simulink model "model_NNMPC_control"  (R2025a)
settings: Solver=ode4  StartTime=0.0  StopTime=100  FixedStep=1  RelTol=1e-4
values from neighbouring files (symbols this model uses):
  q = 0.015    [init_params.m]
  T0 = 320    [init_params.m]
  Tc0 = 298    [init_params.m]
undefined symbols (not defined in the file or in its folder): compactSVM
settings Model: Creator=thapl  LastModifiedBy=thapl
settings DataIOCC: SaveFormat=Array
settings OptimizationCC: ReuseModelBlockBuffer=off
settings RTWCC: GPUComputeCapability=3.5

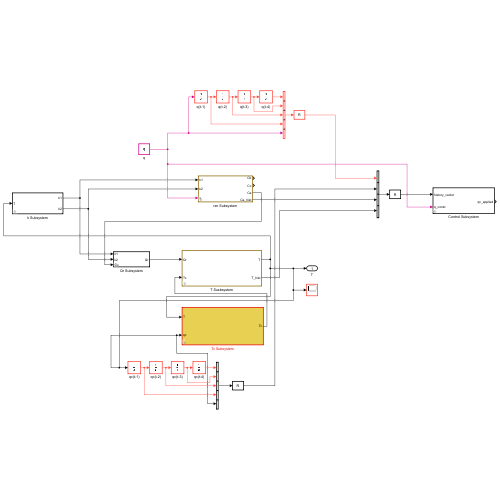
[thumbnail: Simulink's stored preview of the top-level diagram]
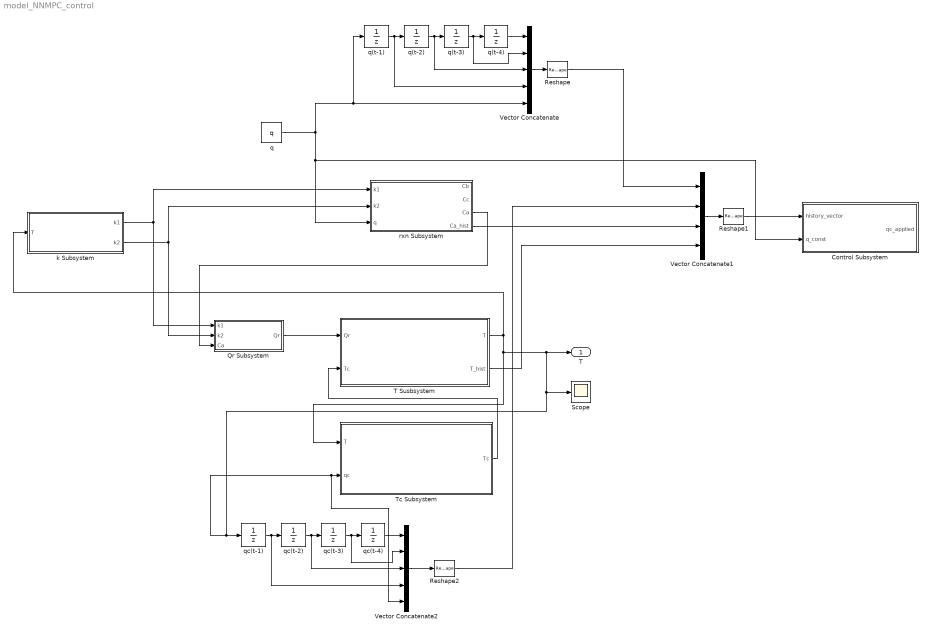
== system model_NNMPC_control ==
  Control Subsystem : Subsystem  mask{T_sp=310}
  Qr Subsystem : Subsystem  mask{V=0.23, dH1=-8.6e4, dH2=-1.82e4}
      mask prompts: V "Reactor Volume (V)"; dH1 "Enthapy of Rxn1 (dH1)"; dH2 "Enthalpy of Rxn2 (dH2)"
  Reshape : Reshape  OutputDimensionality=Customize  OutputDimensions=[1,5]
  Reshape1 : Reshape  OutputDimensionality=Customize  OutputDimensions=[1,20]
  Reshape2 : Reshape  OutputDimensionality=Customize  OutputDimensions=[1,5]
  Scope : Scope
      settings: ActiveDisplayYMinimum=303.48557  ActiveDisplayYMaximum=304.49086
  T Susbsystem : Subsystem  mask{q=0.015, V=0.23, Tf=311, A=1.51, u=42.8, rho=1020, Cp=4.02}
      mask prompts: q "Reactor Flow rate (q)"; V "Reactor Volume (V)"; Tf "Inlet Fluid Temp (Tf)"; A "Contact Area (A)"; u "HTC (u)"; rho "Fluid Density (rho)"; Cp "Specific Heat capactiy (Cp)"
  Tc Subsystem : Subsystem  mask{Vc=0.21, Tcf=292, A=1.51, u=42.8, Cpc=4.182, rhoc=998}
      mask prompts: Vc "Jacket Volume (Vc)"; Tcf "Inlet Cooling Fluid Tempreture (Tcf)"; A "Contact Area (A)"; u "HTC"; Cpc "Specidic Heat Capacity of cooling fluid (Cpc)"; rhoc "Cooling Fluid Density (rhoc)"
  Vector Concatenate : Concatenate  NumInputs=5
  Vector Concatenate1 : Concatenate  NumInputs=4
  Vector Concatenate2 : Concatenate  NumInputs=5
  k Subsystem : Subsystem
      mask DialogControl Control2 Prompt: Text
  q : Constant  Value=q
  q(t-1) : UnitDelay  SampleTime=-1  HasFrameUpgradeWarning=on
  q(t-2) : UnitDelay  SampleTime=-1  HasFrameUpgradeWarning=on
  q(t-3) : UnitDelay  SampleTime=-1  HasFrameUpgradeWarning=on
  q(t-4) : UnitDelay  SampleTime=-1  HasFrameUpgradeWarning=on
  qc(t-1) : UnitDelay  SampleTime=-1  HasFrameUpgradeWarning=on
  qc(t-2) : UnitDelay  SampleTime=-1  HasFrameUpgradeWarning=on
  qc(t-3) : UnitDelay  SampleTime=-1  HasFrameUpgradeWarning=on
  qc(t-4) : UnitDelay  SampleTime=-1  HasFrameUpgradeWarning=on
  rxn Subsystem : Subsystem
      mask DialogControl Control2 Prompt: Reactor
  T : Outport
  wires:
  Tc Subsystem/1(Tc) -> T Susbsystem/2(Tc)
  Qr Subsystem/1(Qr) -> T Susbsystem/1(Qr)
  rxn Subsystem/3(Ca) -> Qr Subsystem/3(Ca)
  k Subsystem/1(k1) -> rxn Subsystem/1(k1), Qr Subsystem/1(k1)
  k Subsystem/2(k2) -> rxn Subsystem/2(k2), Qr Subsystem/2(k2)
  qc(t-2)/1 -> Vector Concatenate2/3, qc(t-3)/1
  qc(t-4)/1 -> Vector Concatenate2/1
  Vector Concatenate2/1 -> Reshape2/1
  qc(t-1)/1 -> Vector Concatenate2/4, qc(t-2)/1
  qc(t-3)/1 -> Vector Concatenate2/2, qc(t-4)/1
  q/1 -> Control Subsystem/2(q_const), rxn Subsystem/3(q), Vector Concatenate/5, q(t-1)/1
  q(t-3)/1 -> Vector Concatenate/2, q(t-4)/1
  q(t-1)/1 -> Vector Concatenate/4, q(t-2)/1
  q(t-4)/1 -> Vector Concatenate/1
  q(t-2)/1 -> Vector Concatenate/3, q(t-3)/1
  Vector Concatenate/1 -> Reshape/1
  rxn Subsystem/4(Ca_hist) -> Vector Concatenate1/3
  Vector Concatenate1/1 -> Reshape1/1
  T Susbsystem/2(T_hist) -> Vector Concatenate1/4
  Reshape/1 -> Vector Concatenate1/1
  Reshape1/1 -> Control Subsystem/1(history_vector)
  Reshape2/1 -> Vector Concatenate1/2
  T Susbsystem/1(T) -> Vector Concatenate2/5, Tc Subsystem/2(qc), qc(t-1)/1, Scope/1, T/1, Tc Subsystem/1(T), k Subsystem/1(T)

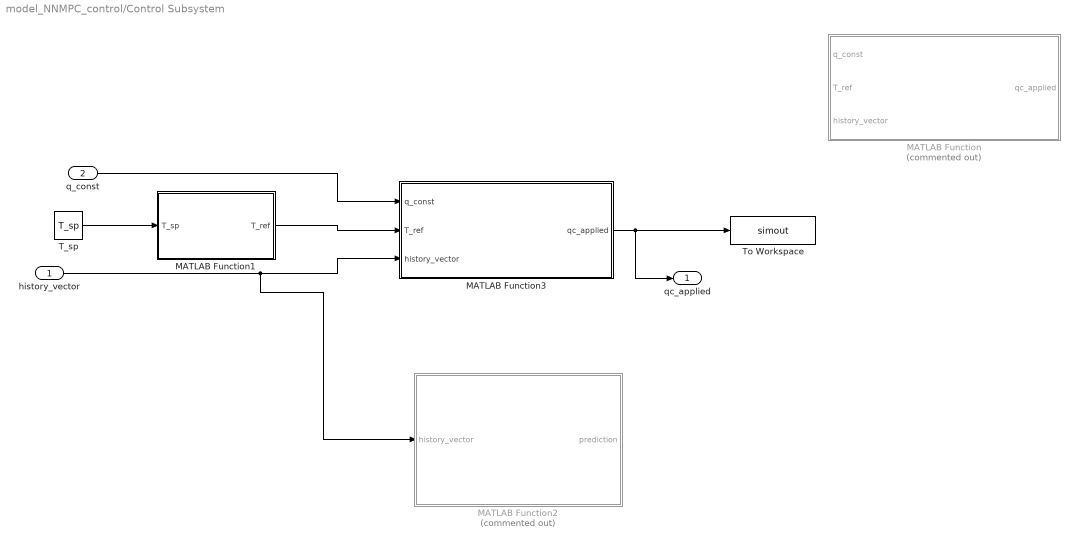
== system model_NNMPC_control/Control Subsystem ==
  history_vector : Inport
  q_const : Inport  Port=2
  MATLAB Function : MATLAB Function  Commented=on  TreatAsAtomicUnit=on  mask{model=compactSVM}
  MATLAB Function1 : MATLAB Function  TreatAsAtomicUnit=on
  MATLAB Function2 : MATLAB Function  Commented=on  TreatAsAtomicUnit=on
  MATLAB Function3 : MATLAB Function  TreatAsAtomicUnit=on
  T_sp : Constant  Value=T_sp
  To Workspace : ToWorkspace  VariableName=simout  SampleTime=-1
      settings: Save2DSignal=2-D array (concatenate along first dimension)
  qc_applied : Outport
  wires:
  T_sp/1 -> MATLAB Function1/1(T_sp)
  history_vector/1 -> MATLAB Function3/3(history_vector), MATLAB Function2/1(history_vector)
  q_const/1 -> MATLAB Function3/1(q_const)
  MATLAB Function1/1(T_ref) -> MATLAB Function3/2(T_ref)
  MATLAB Function3/1(qc_applied) -> qc_applied/1, To Workspace/1

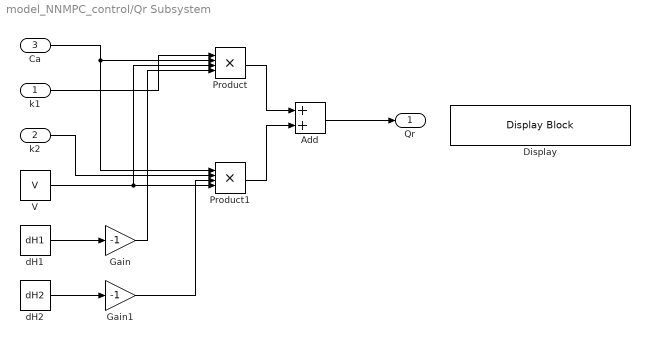
== system model_NNMPC_control/Qr Subsystem ==
  k1 : Inport
  k2 : Inport  Port=2
  Ca : Inport  Port=3
  Add : Sum
  Display : DisplayBlock  LabelPosition=Hide  Transparency=1  GridColor=[0.502, 0.502, 0.502]
  Gain : Gain  Gain=-1
  Gain1 : Gain  Gain=-1
  Product : Product  Inputs=4
  Product1 : Product  Inputs=4
  V : Constant  Value=V
  dH1 : Constant  Value=dH1
  dH2 : Constant  Value=dH2
  Qr : Outport
  wires:
  dH1/1 -> Gain/1
  dH2/1 -> Gain1/1
  k1/1 -> Product/1
  V/1 -> Product1/4, Product/3
  Gain/1 -> Product/4
  Ca/1 -> Product1/1, Product/2
  k2/1 -> Product1/2
  Gain1/1 -> Product1/3
  Product/1 -> Add/1
  Product1/1 -> Add/2
  Add/1 -> Qr/1

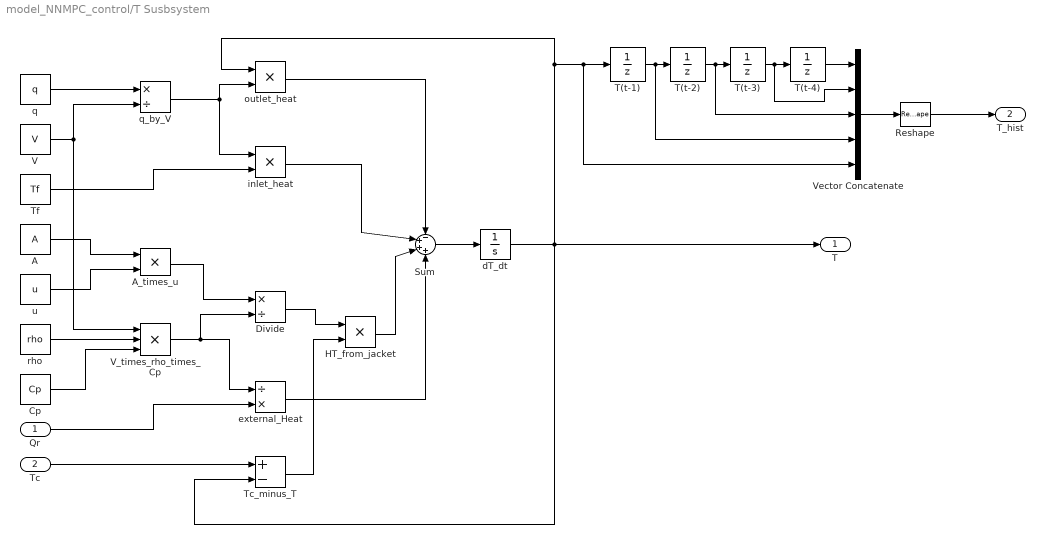
== system model_NNMPC_control/T Susbsystem ==
  Qr : Inport
  Tc : Inport  Port=2
  A : Constant  Value=A
  A_times_u : Product
  Cp : Constant  Value=Cp
  Divide : Product  Inputs=*/
  HT_from_jacket : Product
  Reshape : Reshape  OutputDimensionality=Customize  OutputDimensions=[1,5]
  Sum : Sum  Inputs=-+++
  T(t-1) : UnitDelay  SampleTime=-1  HasFrameUpgradeWarning=on
  T(t-2) : UnitDelay  SampleTime=-1  HasFrameUpgradeWarning=on
  T(t-3) : UnitDelay  SampleTime=-1  HasFrameUpgradeWarning=on
  T(t-4) : UnitDelay  SampleTime=-1  HasFrameUpgradeWarning=on
  Tc_minus_T : Sum  Inputs=+-
  Tf : Constant  Value=Tf
  V : Constant  Value=V
  V_times_rho_times_Cp : Product  Inputs=3
  Vector Concatenate : Concatenate  NumInputs=5
  dT_dt : Integrator  InitialCondition=T0
  external_Heat : Product  Inputs=/*
  inlet_heat : Product
  outlet_heat : Product
  q : Constant  Value=q
  q_by_V : Product  Inputs=*/
  rho : Constant  Value=rho
  u : Constant  Value=u
  T : Outport
  T_hist : Outport  Port=2
  wires:
  q/1 -> q_by_V/1
  V/1 -> V_times_rho_times_Cp/1, q_by_V/2
  q_by_V/1 -> outlet_heat/2, inlet_heat/1
  Tf/1 -> inlet_heat/2
  A/1 -> A_times_u/1
  u/1 -> A_times_u/2
  rho/1 -> V_times_rho_times_Cp/2
  Cp/1 -> V_times_rho_times_Cp/3
  A_times_u/1 -> Divide/1
  V_times_rho_times_Cp/1 -> external_Heat/1, Divide/2
  Divide/1 -> HT_from_jacket/1
  Tc_minus_T/1 -> HT_from_jacket/2
  Qr/1 -> external_Heat/2
  outlet_heat/1 -> Sum/1
  inlet_heat/1 -> Sum/2
  HT_from_jacket/1 -> Sum/3
  external_Heat/1 -> Sum/4
  Sum/1 -> dT_dt/1
  Tc/1 -> Tc_minus_T/1
  dT_dt/1 -> Vector Concatenate/5, T(t-1)/1, outlet_heat/1, T/1, Tc_minus_T/2
  T(t-3)/1 -> Vector Concatenate/2, T(t-4)/1
  T(t-1)/1 -> Vector Concatenate/4, T(t-2)/1
  T(t-4)/1 -> Vector Concatenate/1
  T(t-2)/1 -> Vector Concatenate/3, T(t-3)/1
  Vector Concatenate/1 -> Reshape/1
  Reshape/1 -> T_hist/1

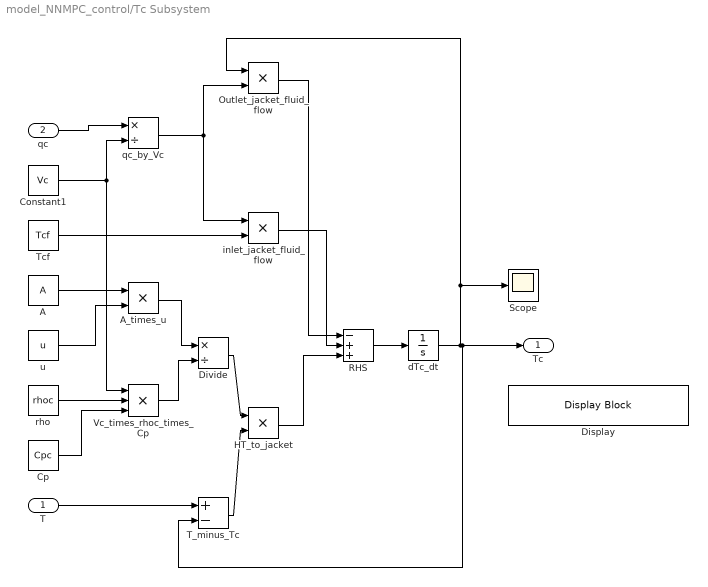
== system model_NNMPC_control/Tc Subsystem ==
  T : Inport
  qc : Inport  Port=2
  A : Constant  Value=A
  A_times_u : Product
  Constant1 : Constant  Value=Vc
  Cp : Constant  Value=Cpc
  Display : DisplayBlock  LabelPosition=Hide  Transparency=1  GridColor=[0.502, 0.502, 0.502]
  Divide : Product  Inputs=*/
  HT_to_jacket : Product
  Outlet_jacket_fluid_flow : Product
  RHS : Sum  Inputs=-++
  Scope : Scope
      settings: ActiveDisplayYMinimum=291.10857  ActiveDisplayYMaximum=300.98794  DataLoggingVariableName=ScopeData3
  T_minus_Tc : Sum  Inputs=+-
  Tcf : Constant  Value=Tcf
  Vc_times_rhoc_times_Cp : Product  Inputs=3
  dTc_dt : Integrator  InitialCondition=Tc0
  inlet_jacket_fluid_flow : Product
  qc_by_Vc : Product  Inputs=*/
  rho : Constant  Value=rhoc
  u : Constant  Value=u
  Tc : Outport
  wires:
  qc/1 -> qc_by_Vc/1
  Constant1/1 -> Vc_times_rhoc_times_Cp/1, qc_by_Vc/2
  qc_by_Vc/1 -> Outlet_jacket_fluid_flow/2, inlet_jacket_fluid_flow/1
  Tcf/1 -> inlet_jacket_fluid_flow/2
  A/1 -> A_times_u/1
  u/1 -> A_times_u/2
  rho/1 -> Vc_times_rhoc_times_Cp/2
  Cp/1 -> Vc_times_rhoc_times_Cp/3
  A_times_u/1 -> Divide/1
  Vc_times_rhoc_times_Cp/1 -> Divide/2
  T/1 -> T_minus_Tc/1
  Divide/1 -> HT_to_jacket/1
  T_minus_Tc/1 -> HT_to_jacket/2
  HT_to_jacket/1 -> RHS/3
  inlet_jacket_fluid_flow/1 -> RHS/2
  RHS/1 -> dTc_dt/1
  dTc_dt/1 -> Scope/1, Outlet_jacket_fluid_flow/1, Tc/1, T_minus_Tc/2
  Outlet_jacket_fluid_flow/1 -> RHS/1

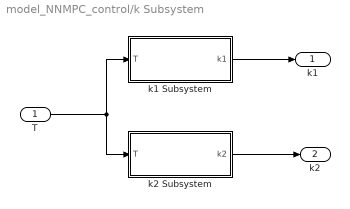
== system model_NNMPC_control/k Subsystem ==
  T : Inport
  k1 Subsystem : Subsystem  mask{R=8.314, k10=1.55e11, Ea1=9850*8.314}
      mask prompts: R "Universal Gas Constant(R)"; k10 "Pre exponential factor(k10)"; Ea1 "Actvation Energy(Ea1)"
  k2 Subsystem : Subsystem  mask{R=8.314, k20=4.55e25, Ea2=22019*8.314}
      mask prompts: R "Universal Gas Constant(R)"; k20 "Pre exponential factor(k10)"; Ea2 "Actvation Energy(Ea1)"
  k1 : Outport
  k2 : Outport  Port=2
  wires:
  k2 Subsystem/1(k2) -> k2/1
  T/1 -> k2 Subsystem/1(T), k1 Subsystem/1(T)
  k1 Subsystem/1(k1) -> k1/1

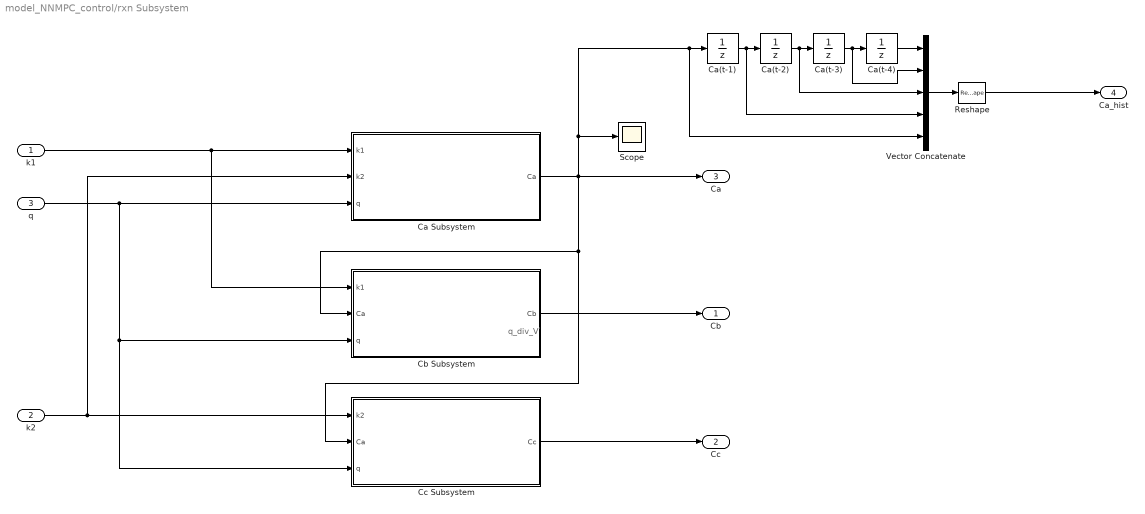
== system model_NNMPC_control/rxn Subsystem ==
  note: q_div_V
  k1 : Inport
  k2 : Inport  Port=2
  q : Inport  Port=3
  Ca Subsystem : Subsystem  mask{V=0.23, Caf=4.22}
      mask prompts: V "Reactor Volume(V)"; Caf "Feed Conc (Caf)"
  Ca(t-1) : UnitDelay  SampleTime=-1  HasFrameUpgradeWarning=on
  Ca(t-2) : UnitDelay  SampleTime=-1  HasFrameUpgradeWarning=on
  Ca(t-3) : UnitDelay  SampleTime=-1  HasFrameUpgradeWarning=on
  Ca(t-4) : UnitDelay  SampleTime=-1  HasFrameUpgradeWarning=on
  Cb Subsystem : Subsystem  mask{V=0.23, Cbf=0}
      mask prompts: V "Reactor Volume(V)"; Cbf "Feed Conc (Cbf)"
  Cc Subsystem : Subsystem  mask{V=0.23, Ccf=0}
      mask prompts: V "Reactor Volume(V)"; Ccf "Feed Conc (Ccf)"
  Reshape : Reshape  OutputDimensionality=Customize  OutputDimensions=[1,5]
  Scope : Scope
      settings: ActiveDisplayYMinimum=3.8625867142774011  ActiveDisplayYMaximum=4.259712587302511
  Vector Concatenate : Concatenate  NumInputs=5
  Cb : Outport
  Cc : Outport  Port=2
  Ca : Outport  Port=3
  Ca_hist : Outport  Port=4
  wires:
  k1/1 -> Cb Subsystem/1(k1), Ca Subsystem/1(k1)
  Cc Subsystem/1(Cc) -> Cc/1
  Cb Subsystem/1(Cb) -> Cb/1
  k2/1 -> Cc Subsystem/1(k2), Ca Subsystem/2(k2)
  q/1 -> Cc Subsystem/3(q), Cb Subsystem/3(q), Ca Subsystem/3(q)
  Ca Subsystem/1(Ca) -> Cc Subsystem/2(Ca), Cb Subsystem/2(Ca), Vector Concatenate/5, Ca(t-1)/1, Scope/1, Ca/1
  Ca(t-3)/1 -> Vector Concatenate/2, Ca(t-4)/1
  Ca(t-1)/1 -> Vector Concatenate/4, Ca(t-2)/1
  Ca(t-4)/1 -> Vector Concatenate/1
  Ca(t-2)/1 -> Vector Concatenate/3, Ca(t-3)/1
  Vector Concatenate/1 -> Reshape/1
  Reshape/1 -> Ca_hist/1

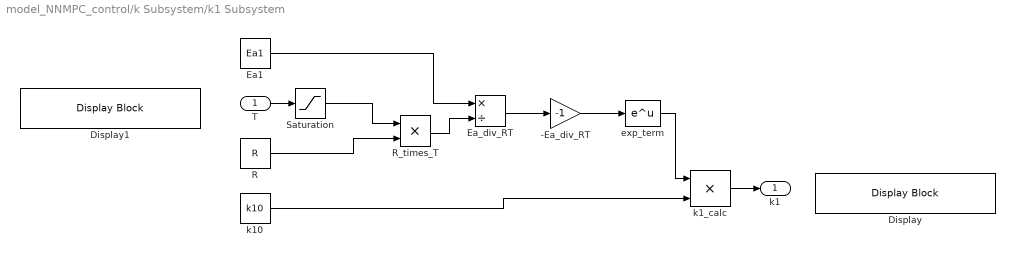
== system model_NNMPC_control/k Subsystem/k1 Subsystem ==
  T : Inport
  -Ea_div_RT : Gain  Gain=-1
  Display : DisplayBlock  LabelPosition=Hide  Transparency=1  GridColor=[0.502, 0.502, 0.502]
  Display1 : DisplayBlock  LabelPosition=Hide  Transparency=1  GridColor=[0.502, 0.502, 0.502]
  Ea1 : Constant  Value=Ea1
  Ea_div_RT : Product  Inputs=*/
  R : Constant  Value=R
  R_times_T : Product
  Saturation : Saturate  UpperLimit=Inf  LowerLimit=0.001
  exp_term : Math
  k10 : Constant  Value=k10
  k1_calc : Product
  k1 : Outport
  wires:
  R/1 -> R_times_T/2
  Ea1/1 -> Ea_div_RT/1
  R_times_T/1 -> Ea_div_RT/2
  k10/1 -> k1_calc/2
  k1_calc/1 -> k1/1
  Ea_div_RT/1 -> -Ea_div_RT/1
  -Ea_div_RT/1 -> exp_term/1
  exp_term/1 -> k1_calc/1
  T/1 -> Saturation/1
  Saturation/1 -> R_times_T/1

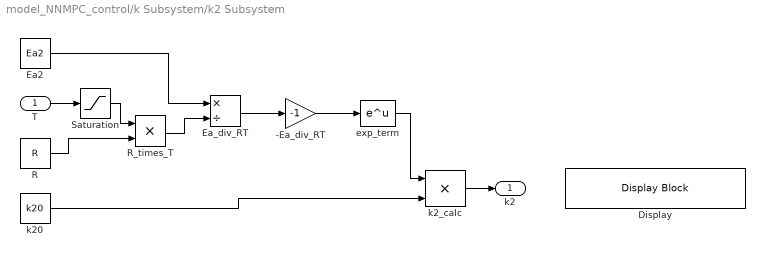
== system model_NNMPC_control/k Subsystem/k2 Subsystem ==
  T : Inport
  -Ea_div_RT : Gain  Gain=-1
  Display : DisplayBlock  LabelPosition=Hide  Transparency=1  GridColor=[0.502, 0.502, 0.502]
  Ea2 : Constant  Value=Ea2
  Ea_div_RT : Product  Inputs=*/
  R : Constant  Value=R
  R_times_T : Product
  Saturation : Saturate  UpperLimit=Inf  LowerLimit=0.001
  exp_term : Math
  k20 : Constant  Value=k20
  k2_calc : Product
  k2 : Outport
  wires:
  R/1 -> R_times_T/2
  Ea2/1 -> Ea_div_RT/1
  R_times_T/1 -> Ea_div_RT/2
  k20/1 -> k2_calc/2
  k2_calc/1 -> k2/1
  Ea_div_RT/1 -> -Ea_div_RT/1
  -Ea_div_RT/1 -> exp_term/1
  exp_term/1 -> k2_calc/1
  T/1 -> Saturation/1
  Saturation/1 -> R_times_T/1

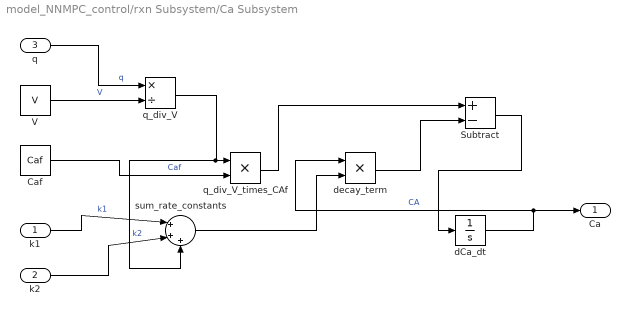
== system model_NNMPC_control/rxn Subsystem/Ca Subsystem ==
  k1 : Inport
  k2 : Inport  Port=2
  q : Inport  Port=3
  Caf : Constant  Value=Caf
  Subtract : Sum  Inputs=+-
  V : Constant  Value=V  SampleTime=Inf
  dCa_dt : Integrator  InitialCondition=4.22
  decay_term : Product
  q_div_V : Product  Inputs=*/
  q_div_V_times_CAf : Product
  sum_rate_constants : Sum  Inputs=|+++
  Ca : Outport
  wires:
  q/1 -> q_div_V/1  "q"
  V/1 -> q_div_V/2  "V"
  q_div_V/1 -> sum_rate_constants/3, q_div_V_times_CAf/1
  Caf/1 -> q_div_V_times_CAf/2  "Caf"
  k1/1 -> sum_rate_constants/1  "k1"
  k2/1 -> sum_rate_constants/2  "k2"
  sum_rate_constants/1 -> decay_term/2
  dCa_dt/1 -> decay_term/1, Ca/1  "CA"
  decay_term/1 -> Subtract/2
  Subtract/1 -> dCa_dt/1
  q_div_V_times_CAf/1 -> Subtract/1

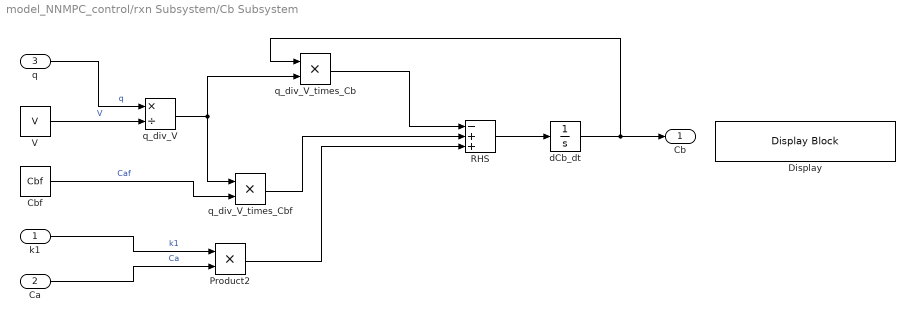
== system model_NNMPC_control/rxn Subsystem/Cb Subsystem ==
  k1 : Inport
  Ca : Inport  Port=2
  q : Inport  Port=3
  Cbf : Constant  Value=Cbf
  Display : DisplayBlock  LabelPosition=Hide  Transparency=1  GridColor=[0.502, 0.502, 0.502]
  Product2 : Product
  RHS : Sum  Inputs=-++
  V : Constant  Value=V
  dCb_dt : Integrator
  q_div_V : Product  Inputs=*/
  q_div_V_times_Cb : Product
  q_div_V_times_Cbf : Product
  Cb : Outport
  wires:
  q/1 -> q_div_V/1  "q"
  V/1 -> q_div_V/2  "V"
  q_div_V/1 -> q_div_V_times_Cb/2, q_div_V_times_Cbf/1
  Cbf/1 -> q_div_V_times_Cbf/2  "Caf"
  k1/1 -> Product2/1  "k1"
  dCb_dt/1 -> Cb/1, q_div_V_times_Cb/1
  RHS/1 -> dCb_dt/1
  Ca/1 -> Product2/2  "Ca"
  q_div_V_times_Cb/1 -> RHS/1
  q_div_V_times_Cbf/1 -> RHS/2
  Product2/1 -> RHS/3

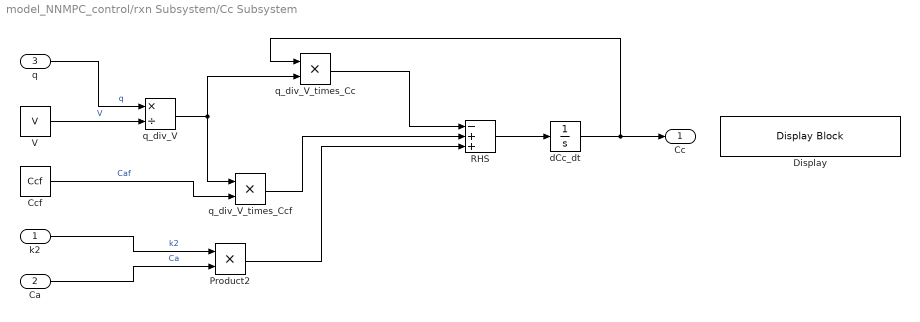
== system model_NNMPC_control/rxn Subsystem/Cc Subsystem ==
  k2 : Inport
  Ca : Inport  Port=2
  q : Inport  Port=3
  Ccf : Constant  Value=Ccf
  Display : DisplayBlock  LabelPosition=Hide  Transparency=1  GridColor=[0.502, 0.502, 0.502]
  Product2 : Product
  RHS : Sum  Inputs=-++
  V : Constant  Value=V
  dCc_dt : Integrator
  q_div_V : Product  Inputs=*/
  q_div_V_times_Cc : Product
  q_div_V_times_Ccf : Product
  Cc : Outport
  wires:
  q/1 -> q_div_V/1  "q"
  V/1 -> q_div_V/2  "V"
  q_div_V/1 -> q_div_V_times_Cc/2, q_div_V_times_Ccf/1
  Ccf/1 -> q_div_V_times_Ccf/2  "Caf"
  k2/1 -> Product2/1  "k2"
  dCc_dt/1 -> Cc/1, q_div_V_times_Cc/1
  RHS/1 -> dCc_dt/1
  Ca/1 -> Product2/2  "Ca"
  q_div_V_times_Cc/1 -> RHS/1
  q_div_V_times_Ccf/1 -> RHS/2
  Product2/1 -> RHS/3

== matlab function model_NNMPC_control/Control Subsystem/MATLAB Function1 ==
  data: T_sp input; T_ref output
function T_ref  = fcn(T_sp)

% Define fixed-size output vectors
T_ref = zeros(1,10);

T_ref(:) = T_sp;

end

== matlab function model_NNMPC_control/Control Subsystem/MATLAB Function ==
  data: q_const input; qc_applied output; T_ref input; history_vector input
function qc_applied = NN_MPC_Controller(q_const, T_ref,history_vector )
% Inputs:
%   history_vector: 1x20 vector [q_hist, qc_hist, T_hist, Ca_hist]
%   T_ref: 1xP desired future temperatures
%   q_const: scalar assumed constant q for future steps
% Output:
%   qc_applied: scalar coolant input to apply

    P = length(T_ref);           
    lambda = 1.0;                 
    qc_prev = history_vector(10); 

    q_seq = repmat(q_const, 1, P);

    qc0 = repmat(qc_prev, 1, P);
    lb = zeros(1, P);
    ub = repmat(0.03, 1, P);

    costFcn = @(qc_seq) costWrapper(qc_seq, history_vector, q_seq, qc_prev, T_ref, lambda);

    options = optimoptions('fmincon','Display','none','Algorithm','sqp');
    [qc_opt, ~] = fmincon(costFcn, qc0, [], [], [], [], lb, ub, [], options);

    qc_applied = qc_opt(1);
end

function [T_preds, Ca_preds] = predictRolling_vector(history_vector, qc_seq, q_seq)
    P = length(qc_seq);
    T_preds = zeros(1, P);
    Ca_preds = zeros(1, P);

    q_hist  = history_vector(1:5);
    qc_hist = history_vector(6:10);
    T_hist  = history_vector(11:15);
    Ca_hist = history_vector(16:20);

    for i = 1:P
        input_vector = [q_hist, qc_hist, T_hist, Ca_hist];
        output = RegressionPredict( input_vector); 
        T_preds(i) = output(1);
        Ca_preds(i) = output(2);

        q_hist  = [q_hist(2:end), q_seq(i)];
        qc_hist = [qc_hist(2:end), qc_seq(i)];
        T_hist  = [T_hist(2:end), T_preds(i)];
        Ca_hist = [Ca_hist(2:end), Ca_preds(i)];
    end
end

function J = costWrapper(qc_seq, history_vector, q_seq, qc_prev, T_ref, lambda)

    [T_preds, ~] = predictRolling_vector(history_vector, qc_seq, q_seq);

    tracking_error = sum((T_preds - T_ref).^2);
    delta_qc = diff([qc_prev, qc_seq]);
    effort = sum(delta_qc.^2);

    J = tracking_error + lambda * effort;
end

function predictions = RegressionPredict(InputData)
%#codegen
    persistent model
    if isempty(model)
        tmp = load('trainedModel.mat');  % Ensure this file is saved in the workspace
        model = tmp.trainedModel;
    end

    % Convert the input vector to a table with proper variable names
    inputTable = array2table(InputData, 'VariableNames', model.RequiredVariables);

    % Predict using the model's predict function
    predictions = model.predictFcn(inputTable);

    % If the model returns a table or struct, unpack it here if needed
    % predictions = [predictions.T, predictions.Ca];  % Example, if model returns a struct
end

== matlab function model_NNMPC_control/Control Subsystem/MATLAB Function2 ==
  settings: updateMethod=DISCRETE
  data: history_vector input; prediction output
function prediction = predictOutput(history_vector)
%#codegen

% Explicitly declare output size and type for Simulink inference
% Input: 1x20 single
% Output: 1x2 single
prediction = zeros(1, 2, 'single');

% Load the network only once
persistent net; %#ok<NASGU>
if isempty(net)
    net = coder.loadDeepLearningNetwork("trainedOnnxNet.mat", "net");
end

% Predict output using the loaded network
prediction = predict(net, history_vector);

end

== matlab function model_NNMPC_control/Control Subsystem/MATLAB Function3 ==
  settings: updateMethod=DISCRETE
  data: q_const input; qc_applied output; T_ref input; history_vector input
function qc_applied = NN_MPC_Controller(q_const, T_ref, history_vector)
%#codegen
    P = length(T_ref);
    lambda = 1.0;
    qc_prev = history_vector(10);
    q_seq = repmat(q_const, 1, P);
    qc0 = repmat(qc_prev, 1, P);
    lb = zeros(1, P);
    ub = repmat(0.03, 1, P);
    
    % Create options without Display (not supported in codegen)
    options = optimoptions('fmincon','Algorithm','sqp','MaxIterations',100,'OptimalityTolerance',1e-6);
    
    % Call the wrapper function with explicit parameters
    [qc_opt, ~] = myFminconWrapper_Alternative(qc0, lb, ub, options, history_vector, q_seq, qc_prev, T_ref, lambda);
    qc_applied = qc_opt(1);
end

function [T_preds, Ca_preds] = predictRolling_vector(history_vector, qc_seq, q_seq)
%#codegen
    P = length(qc_seq);
    T_preds = zeros(1, P);
    Ca_preds = zeros(1, P);
    
    q_hist = history_vector(1:5);
    qc_hist = history_vector(6:10);
    T_hist = history_vector(11:15);
    Ca_hist = history_vector(16:20);
    
    for i = 1:P
        input_vector = [q_hist, qc_hist, T_hist, Ca_hist];
        output = predictOutput(input_vector);
        T_preds(i) = output(1);
        Ca_preds(i) = output(2);
        
        q_hist = [q_hist(2:end), q_seq(i)];
        qc_hist = [qc_hist(2:end), qc_seq(i)];
        T_hist = [T_hist(2:end), T_preds(i)];
        Ca_hist = [Ca_hist(2:end), Ca_preds(i)];
    end
end

function prediction = predictOutput(history_vector)
%#codegen
    % Explicitly declare output size and type for Simulink inference
    prediction = zeros(1, 2, 'single');
    
    % Load the network only once
    persistent net;
    if isempty(net)
        net = coder.loadDeepLearningNetwork("trainedOnnxNet.mat", "net");
    end
    
    % Predict output using the loaded network
    prediction = predict(net, history_vector);
end

% Method 1: Using global variables (Simulink-compatible approach)
function [qc_opt, Jval] = myFminconWrapper(qc0, lb, ub, options, history_vector, q_seq, qc_prev, T_ref, lambda)
%#codegen
    % Store parameters in persistent variables to avoid function handle issues
    persistent p_history_vector p_q_seq p_qc_prev p_T_ref p_lambda;
    
    p_history_vector = history_vector;
    p_q_seq = q_seq;
    p_qc_prev = qc_prev;
    p_T_ref = T_ref;
    p_lambda = lambda;
    
    % Use string function name instead of function handle
    [qc_opt, Jval] = fmincon('costFcnPersistent', qc0, [], [], [], [], lb, ub, [], options);
end

% Cost function that uses persistent variables
function J = costFcnPersistent(qc_seq)
%#codegen
    persistent p_history_vector p_q_seq p_qc_prev p_T_ref p_lambda;
    
    % Check if persistent variables are initialized
    if isempty(p_history_vector)
        J = inf; % Return large value if not initialized
        return;
    end
    
    [T_preds, ~] = predictRolling_vector(p_history_vector, qc_seq, p_q_seq);
    tracking_error = sum((T_preds - p_T_ref).^2);
    delta_qc = diff([p_qc_prev, qc_seq]);
    effort = sum(delta_qc.^2);
    J = tracking_error + p_lambda * effort;
end

% Method 2: Alternative approach using optimization problem structure
function [qc_opt, Jval] = myFminconWrapper_Alternative(qc0, lb, ub, options, history_vector, q_seq, qc_prev, T_ref, lambda)
%#codegen
    % For Simulink, we might need to use a simpler optimization approach
    % This implements a basic gradient descent as fallback
    
    qc_opt = qc0;
    learning_rate = 0.01;
    max_iter = 50;
    tolerance = 1e-6;
    
    for iter = 1:max_iter
        % Evaluate current cost
        J_current = costFcnStandalone(qc_opt, history_vector, q_seq, qc_prev, T_ref, lambda);
        
        % Compute numerical gradient
        grad = zeros(size(qc_opt));
        epsilon = 1e-6;
        
        for i = 1:length(qc_opt)
            qc_plus = qc_opt;
            qc_plus(i) = qc_plus(i) + epsilon;
            J_plus = costFcnStandalone(qc_plus, history_vector, q_seq, qc_prev, T_ref, lambda);
            grad(i) = (J_plus - J_current) / epsilon;
        end
        
        % Update with gradient descent
        qc_new = qc_opt - learning_rate * grad;
        
        % Apply bounds
        qc_new = max(lb, min(ub, qc_new));
        
        % Check convergence
        if norm(qc_new - qc_opt) < tolerance
            break;
        end
        
        qc_opt = qc_new;
    end
    
    Jval = costFcnStandalone(qc_opt, history_vector, q_seq, qc_prev, T_ref, lambda);
end

% Method 3: Simple iterative optimization for Simulink compatibility
function [qc_opt, Jval] = myFminconWrapper_Simple(qc0, lb, ub, options, history_vector, q_seq, qc_prev, T_ref, lambda)
%#codegen
    % Use a pattern search approach that's more Simulink-friendly
    qc_opt = qc0;
    best_cost = costFcnStandalone(qc0, history_vector, q_seq, qc_prev, T_ref, lambda);
    
    % Simple pattern search
    step_size = 0.001;
    num_iterations = 30;
    
    for iter = 1:num_iterations
        improved = false;
        
        for i = 1:length(qc_opt)
            % Try positive step
            qc_test = qc_opt;
            qc_test(i) = min(ub(i), qc_test(i) + step_size);
            cost_test = costFcnStandalone(qc_test, history_vector, q_seq, qc_prev, T_ref, lambda);
            
            if cost_test < best_cost
                qc_opt = qc_test;
                best_cost = cost_test;
                improved = true;
                continue;
            end
            
            % Try negative step
            qc_test = qc_opt;
            qc_test(i) = max(lb(i), qc_test(i) - step_size);
            cost_test = costFcnStandalone(qc_test, history_vector, q_seq, qc_prev, T_ref, lambda);
            
            if cost_test < best_cost
                qc_opt = qc_test;
                best_cost = cost_test;
                improved = true;
            end
        end
        
        if ~improved
            step_size = step_size * 0.5; % Reduce step size
            if step_size < 1e-6
                break;
            end
        end
    end
    
    Jval = best_cost;
end

% Standalone cost function (keep this unchanged)
function J = costFcnStandalone(qc_seq, history_vector, q_seq, qc_prev, T_ref, lambda)
%#codegen
    [T_preds, ~] = predictRolling_vector(history_vector, qc_seq, q_seq);
    tracking_error = sum((T_preds - T_ref).^2);
    delta_qc = diff([qc_prev, qc_seq]);
    effort = sum(delta_qc.^2);
    J = tracking_error + lambda * effort;
end
